simulink model "STOICAL_example_1_Step00_ExistingModel"  (R2014b)
settings: Solver=ode4  StartTime=0.0  StopTime=1  FixedStep=50E-6  RelTol=1e-3
settings Model: Creator=Wippenbeck  LastModifiedBy=Wippenbeck

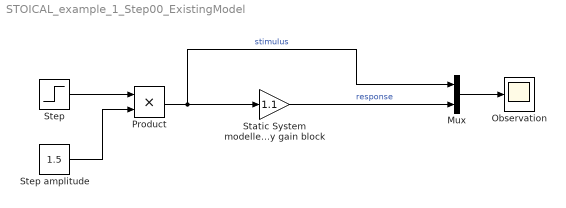
== system STOICAL_example_1_Step00_ExistingModel ==
  Mux : Mux  Inputs=2
  Observation : Scope
      settings: ShowLegends=on  TimeRange=1  YMin=0  YMax=1
  Product : Product
  Static System modelled by gain block : Gain  Gain=1.1
  Step : Step  Time=0.1  SampleTime=0
  Step amplitude : Constant  Value=1.5
  wires:
  Product/1 -> Static System modelled by gain block/1, Mux/1  "stimulus"
  Static System modelled by gain block/1 -> Mux/2  "response"
  Mux/1 -> Observation/1
  Step/1 -> Product/1
  Step amplitude/1 -> Product/2
